simulink model "ZynqBallTrackerFPGA"  (R2017a)
settings: Solver=FixedStepDiscrete  StartTime=0.0  StopTime=5.0  RelTol=1e-3  EnableMultiTasking=on
PostLoadFcn:
  | model_init
values from neighbouring files (symbols this model uses):
  C = 1920    [model_init.m]
  HueTarg = 150    [model_init.m]
  HueTol = 20    [model_init.m]
  Kd = 1    [model_init.m]
  KernG_hdl = reshape(KernG,[],1)    [model_init.m]
  KernR1B2_hdl = reshape(KernR1B2,[],1)    [model_init.m]
  KernR2B1_hdl = reshape(KernR2B1,[],1)    [model_init.m]
  KernRB_hdl = reshape(KernRB,[],1)    [model_init.m]
  Ki = 4    [model_init.m]
  Kp = 16    [model_init.m]
  P = polyfit(u,y,N)    [calc_gamma.m]    (also in model_init.m = calc_gamma(GammaErr,3))
  PWM_CNT = 1024e3    (= 1024000)    [model_init.m]
  R = 1080    [model_init.m]
  SatTarg = 0.38    [model_init.m]
  SatTol = 0.05    [model_init.m]
  SaturationLimit = 256    [model_init.m]
  TsFPGA = TsFr/(R*C)    (= 1.60751028807e-08)    [model_init.m]
  TsFr = 1/FrRt    (= 0.0333333333333)    [model_init.m]
  ValTarg = 170    [model_init.m]
  ValTol = 45    [model_init.m]
undefined symbols (not defined in the file or in its folder): gray, Rec, SDTV
libraries: hdlsllib x51, simulink x12, simulink_need_slupdate x10, visionconversions x2, visiontextngfix x2, visionstatistics x1, dspvision x1, visiongeotforms x1, dspsigattribs x1, dspbuff3 x1
(part 1 of 2)
settings Model: SimulationMode=accelerator  Creator=mfornero  LastModifiedBy=skuznick
settings DataIOCC: LimitDataPoints=on  SaveFormat=Array
settings OptimizationCC: BlockReduction=off  ConditionallyExecuteInputs=off  DefaultParameterBehavior=Inlined  LifeSpan=inf
settings DebuggingCC: AlgebraicLoopMsg=error  UnderspecifiedInitializationDetection=Classic  MergeDetectMultiDrivingBlocksExec=none  InheritedTsInSrcMsg=none  SFUnexpectedBacktrackingDiag=warning  SFNoUnconditionalDefaultTransitionDiag=warning  SFExecutionAtInitializationDiag=none
settings HardwareCC: ProdBitPerPointer=32  ProdBitPerSizeT=32  ProdBitPerPtrDiffT=32  ProdLargestAtomicFloat=None  ProdIntDivRoundTo=Undefined  ProdEndianess=Unspecified  ProdWordSize=32  ProdHWDeviceType=ASIC/FPGA->ASIC/FPGA  ProdEqTarget=off
settings ModelReferenceCC: PropagateSignalLabelsOutOfModel=off
settings GRTTargetCC: TargetLangStandard=C89/C90 (ANSI)  GeneratePreprocessorConditionals=Disable all
settings ConfigComp: CovMetricSettings=dw  CovHtmlReporting=on  CovSaveCumulativeToWorkspaceVar=on  CovSaveSingleToWorkspaceVar=on  CovExternalEMLEnable=off  CovSFcnEnable=off

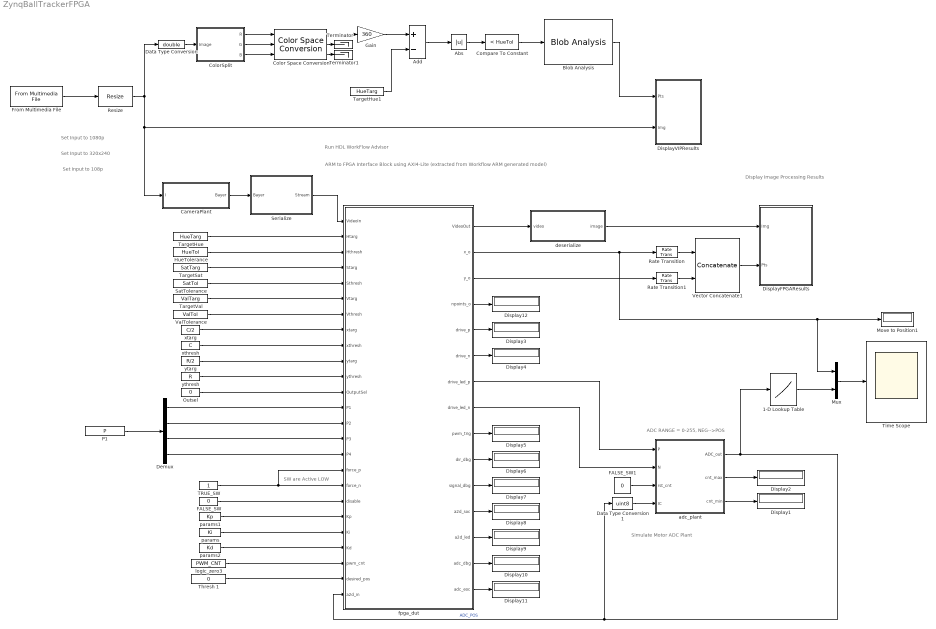
== system ZynqBallTrackerFPGA ==
  note: Set Input to 1080p
  note: Set Input to 320x240
  note: Set Input to 108p
  note: ADC RANGE = 0-255, NEG-->POS
  note: Simulate Motor ADC Plant
  note: Display Image Processing
      | Results
  note: SW are Active LOW
  note: ARM to FPGA Interface Block
      | using AXI4-Lite (extracted from Workflow ARM generated model)
  note: Run HDL WorkFlow
      | Advisor
  1-D Lookup Table : Lookup_n-D  NumberOfTableDimensions=1  BreakpointsForDimension1=[0:1:255]  IndexSearchMethod=Evenly spaced points  Table=[254:-2:-256]  TableDataTypeStr=Inherit: Inherit from 'Table data'  InterpMethod=Flat  DiagnosticForOutOfRangeInput=Error  OutDataTypeStr=fixdt(0,32,0)  RndMeth=Simplest  InputSameDT=on
  Abs : Abs
  Add : Sum  Inputs=+-
  Blob Analysis : visionstatistics/Blob Analysis  Tag=vipblks_row_conv  area=off  centroid=on  bBox=off  majorAxis=off  minorAxis=off  angle=off  eccentricity=off  equivDiameterSq=off  extent=off  perimeter=off  maxBlobs=1  warnIfNumBlobsExceeded=off  isCount=off  useMinArea=on  minArea=100  useMaxArea=off  maxArea=intmax('uint32')  excludeBorderBlob=on  outDT=Specify via Data Types tab  isOutVarDim=off  isFill=off  fillValues=-1  conn=4  isLabel=off  outputMode=Binary point scaling  outputWordLength=16  outputFracLength=0  firstCoeffMode=Binary point scaling  firstCoeffWordLength=16  firstCoeffFracLength=14  secondCoeffMode=Binary point scaling  secondCoeffWordLength=32  secondCoeffFracLength=16  accumMode=Binary point scaling  accumWordLength=32  accumFracLength=0  prodOutputMode=Binary point scaling  prodOutputWordLength=32  prodOutputFracLength=16  roundingMode=Floor  overflowMode=off
      settings: SourceProductName=Computer Vision System Toolbox
  CameraPlant : Subsystem
  Color Space Conversion : visionconversions/Color Space  Conversion  conversion=Obsolete  conversionActive=R'G'B' to HSV  wp_str=D65  rec=Rec. 601 (SDTV)  sys=1125/60/2:1  imagePorts=Separate color signals
      settings: SourceProductName=Computer Vision System Toolbox
  ColorSplit : Subsystem
  Compare To Constant : simulink/Logic and Bit Operations/Compare To Constant  relop=<  const=HueTol  OutDataTypeStr=boolean
  Data Type Conversion : DataTypeConversion  OutDataTypeStr=double
  Data Type Conversion1 : DataTypeConversion  OutDataTypeStr=uint8
  Demux : Demux
  Display{1..12} (12 alike) : Display
  DisplayFPGAResults : Subsystem
  DisplayVIPResults : Subsystem
  FALSE_SW : Constant  Value=0  OutDataTypeStr=boolean  SampleTime=-1
  FALSE_SW1 : Constant  Value=0  OutDataTypeStr=boolean  SampleTime=-1
  From Multimedia File : dspvision/From Multimedia File  inputFilename=Ball.wmv  loop=on  numPlays=inf  outputStreams=Video only  videoDataType=uint8  audioDataType=int16  inheritSampleTime=off  userDefinedSampleTime=TsFr  noAudioOutput=off  isIntensityVideo=off  fourcc=RGB  colorVideoFormat=One multidimensional signal  outputEOF=off  dataOrg=Column-major  audioFrameSize=1024  computeAudioFrameSize=off  outSamplingMode=Frame based
      settings: SourceProductBaseCode=VP
  Gain : Gain  Gain=360
  "HueTolerance " : Constant  Value=HueTol  OutDataTypeStr=Inherit: Inherit via back propagation  SampleTime=-1
  Move to Position1 : Display
  Mux : Mux  Inputs=2
  Outsel : Constant  Value=0  OutDataTypeStr=Inherit: Inherit via back propagation  SampleTime=-1
  P1 : Constant  Value=P  OutDataTypeStr=fixdt(1,25,22)  SampleTime=-1
  Rate Transition : RateTransition  OutPortSampleTime=TsFr
  Rate Transition1 : RateTransition  OutPortSampleTime=TsFr
  Resize : visiongeotforms/Resize  specify=Number of output rows and columns  rfactor=[200 150]  outCols=25  outRows=25  outRowsCols=[R C]  interp_method=Bilinear  antialias=on  useROI=off  roiFlag=off  prodOutputMode=Binary point scaling  prodOutputWordLength=32  prodOutputFracLength=10  roundingMode=Nearest  overflowMode=on
      settings: SourceProductName=Computer Vision System Toolbox  SourceProductBaseCode=VP
  SatTolerance : Constant  Value=SatTol  OutDataTypeStr=Inherit: Inherit via back propagation  SampleTime=-1
  Serialize : Subsystem
  TRUE_SW : Constant  OutDataTypeStr=boolean  SampleTime=-1
  TargetHue : Constant  Value=HueTarg  OutDataTypeStr=Inherit: Inherit via back propagation  SampleTime=-1
  TargetHue1 : Constant  Value=HueTarg  OutDataTypeStr=Inherit: Inherit via back propagation  SampleTime=-1
  TargetSat : Constant  Value=SatTarg  OutDataTypeStr=Inherit: Inherit via back propagation  SampleTime=-1
  TargetVal : Constant  Value=ValTarg  OutDataTypeStr=Inherit: Inherit via back propagation  SampleTime=-1
  Terminator : Terminator
  Terminator1 : Terminator
  Thresh 1 : Constant  Value=0  OutDataTypeStr=Inherit: Inherit via back propagation  SampleTime=-1
  Time Scope : Scope
  ValTolerance : Constant  Value=ValTol  OutDataTypeStr=Inherit: Inherit via back propagation  SampleTime=-1
  Vector Concatenate1 : Concatenate  Mode=Multidimensional array  ConcatenateDimension=2
  adc_plant : Subsystem
  deserialize : Subsystem
  fpga_dut : Subsystem  TreatAsAtomicUnit=on
  logic_zero3 : Constant  Value=PWM_CNT  OutDataTypeStr=fixdt(0,22,0)  SampleTime=-1
  params : Constant  Value=Ki  OutDataTypeStr=fixdt(1,20,14)  SampleTime=-1
  params1 : Constant  Value=Kp  OutDataTypeStr=fixdt(1,20,14)  SampleTime=-1
  params2 : Constant  Value=Kd  OutDataTypeStr=fixdt(1,20,14)  SampleTime=-1
  xtarg : Constant  Value=C/2  OutDataTypeStr=Inherit: Inherit via back propagation  SampleTime=-1
  xthresh : Constant  Value=C  OutDataTypeStr=Inherit: Inherit via back propagation  SampleTime=-1
  ytarg : Constant  Value=R/2  OutDataTypeStr=Inherit: Inherit via back propagation  SampleTime=-1
  ythresh : Constant  Value=R  OutDataTypeStr=Inherit: Inherit via back propagation  SampleTime=-1
  wires:
  From Multimedia File/1 -> Resize/1
  Resize/1 -> CameraPlant/1(I), DisplayVIPResults/2(Img), Data Type Conversion/1
  Blob Analysis/1 -> DisplayVIPResults/1(Pts)
  Data Type Conversion/1 -> ColorSplit/1(Image)
  Serialize/1(Stream) -> fpga_dut/1(VideoIn)
  TargetHue/1 -> fpga_dut/2(Htarg)
  Outsel/1 -> fpga_dut/12(OutputSel)
  "HueTolerance "/1 -> fpga_dut/3(Hthresh)
  fpga_dut/1(VideoOut) -> deserialize/1(video)
  deserialize/1(image) -> DisplayFPGAResults/1(Img)
  ColorSplit/2(G) -> Color Space Conversion/2
  ColorSplit/3(B) -> Color Space Conversion/3
  ColorSplit/1(R) -> Color Space Conversion/1
  Abs/1 -> Compare To Constant/1
  Color Space Conversion/1 -> Gain/1
  Add/1 -> Abs/1
  TargetHue1/1 -> Add/2
  Gain/1 -> Add/1
  Color Space Conversion/2 -> Terminator/1
  Color Space Conversion/3 -> Terminator1/1
  Compare To Constant/1 -> Blob Analysis/1
  Demux/2 -> fpga_dut/14(P2)
  Demux/3 -> fpga_dut/15(P3)
  Demux/1 -> fpga_dut/13(P1)
  Demux/4 -> fpga_dut/16(P4)
  P1/1 -> Demux/1
  CameraPlant/1(Bayer) -> Serialize/1(Bayer)
  TargetSat/1 -> fpga_dut/4(Starg)
  SatTolerance/1 -> fpga_dut/5(Sthresh)
  TargetVal/1 -> fpga_dut/6(Vtarg)
  ValTolerance/1 -> fpga_dut/7(Vthresh)
  adc_plant/2(cnt_max) -> Display2/1
  adc_plant/3(cnt_min) -> Display1/1
  adc_plant/1(ADC_out) -> Data Type Conversion1/1, fpga_dut/25(a2d_in), 1-D Lookup Table/1  "ADC_POS"
  Data Type Conversion1/1 -> adc_plant/4(IC)
  Mux/1 -> Time Scope/1
  fpga_dut/7(drive_led_p) -> adc_plant/1(P)
  fpga_dut/8(drive_led_n) -> adc_plant/2(N)
  FALSE_SW1/1 -> adc_plant/3(rst_cnt)
  1-D Lookup Table/1 -> Mux/2
  fpga_dut/2(x_o) -> Rate Transition/1, Mux/1, Move to Position1/1
  Rate Transition/1 -> Vector Concatenate1/1
  Rate Transition1/1 -> Vector Concatenate1/2
  Vector Concatenate1/1 -> DisplayFPGAResults/2(Pts)
  fpga_dut/3(y_o) -> Rate Transition1/1
  fpga_dut/5(drive_p) -> Display3/1
  fpga_dut/6(drive_n) -> Display4/1
  fpga_dut/9(pwm_trig) -> Display5/1
  fpga_dut/10(dir_dbg) -> Display6/1
  fpga_dut/11(signal_dbg) -> Display7/1
  fpga_dut/12(a2d_soc) -> Display8/1
  fpga_dut/13(a2d_led) -> Display9/1
  fpga_dut/14(adc_dbg) -> Display10/1
  fpga_dut/15(adc_eoc) -> Display11/1
  TRUE_SW/1 -> fpga_dut/17(force_p), fpga_dut/18(force_n)
  FALSE_SW/1 -> fpga_dut/19(disable)
  params/1 -> fpga_dut/21(Ki)
  params1/1 -> fpga_dut/20(Kp)
  params2/1 -> fpga_dut/22(Kd)
  logic_zero3/1 -> fpga_dut/23(pwm_cnt)
  Thresh 1/1 -> fpga_dut/24(desired_pos)
  xtarg/1 -> fpga_dut/8(xtarg)
  xthresh/1 -> fpga_dut/9(xthresh)
  ytarg/1 -> fpga_dut/10(ytarg)
  ythresh/1 -> fpga_dut/11(ythresh)
  fpga_dut/4(npoints_o) -> Display12/1

== system ZynqBallTrackerFPGA/CameraPlant ==
  I : Inport
  Bayer_Phase1 : Constant  Value=3  SampleTime=TsFr
  Gamma Correction VIP : visionconversions/Gamma Correction  operation=De-gamma  gamma=GammaErr  linearSegment=off  breakPoint=0.018
      settings: SourceProductName=Computer Vision System Toolbox  SourceProductBaseCode=VP
  mosaic : MATLAB Function  TreatAsAtomicUnit=on
  Bayer : Outport
  wires:
  Bayer_Phase1/1 -> mosaic/2(phase)
  mosaic/1(Y) -> Bayer/1
  I/1 -> Gamma Correction VIP/1
  Gamma Correction VIP/1 -> mosaic/1(I)

== system ZynqBallTrackerFPGA/ColorSplit ==
  Image : Inport
  SelB : Selector  NumberOfDimensions=3  InputPortWidth=5  IndexOptions=Select all,Select all,Index vector (dialog)  Indices=[1],1,3  OutputSizes=1,1,1
  SelG : Selector  NumberOfDimensions=3  InputPortWidth=5  IndexOptions=Select all,Select all,Index vector (dialog)  Indices=[1],1,2  OutputSizes=1,1,1
  SelR : Selector  NumberOfDimensions=3  InputPortWidth=5  IndexOptions=Select all,Select all,Index vector (dialog)  Indices=[1],1,1  OutputSizes=1,1,1
  R : Outport
  G : Outport  Port=2
  B : Outport  Port=3
  wires:
  SelR/1 -> R/1
  SelG/1 -> G/1
  Image/1 -> SelB/1, SelR/1, SelG/1
  SelB/1 -> B/1

== system ZynqBallTrackerFPGA/DisplayFPGAResults ==
  Img : Inport
  Pts : Inport  Port=2
  Draw Markers : visiontextngfix/Draw Markers  shape=Circle  size=msize  fill=on  fillClrSource=Specify via dialog  display=User-specified value  intensity=200  color=[255 0 0]  opacity=1.0  viewport=Entire image  antialiasing=off  inType=Obsolete  imagePorts=One multidimensional signal  prodOutputMode=Binary point scaling  prodOutputWordLength=32  prodOutputFracLength=14  memoryMode=Specify word length  memoryWordLength=16  memoryFracLength=14  roundingMode=Floor  overflowMode=off
      settings: SourceProductName=Computer Vision System Toolbox  SourceProductBaseCode=VP
  FPGAViewer : VideoViewer  colormapValue=gray(256)  FigPos=[562 1008 521 308]
  wires:
  Img/1 -> Draw Markers/1
  Pts/1 -> Draw Markers/2
  Draw Markers/1 -> FPGAViewer/1

== system ZynqBallTrackerFPGA/DisplayVIPResults ==
  Pts : Inport
  Img : Inport  Port=2
  Draw Markers : visiontextngfix/Draw Markers  shape=Circle  size=msize  fill=on  fillClrSource=Specify via dialog  display=User-specified value  intensity=200  color=[255 0 0]  opacity=1.0  viewport=Entire image  antialiasing=off  inType=Obsolete  imagePorts=One multidimensional signal  prodOutputMode=Binary point scaling  prodOutputWordLength=32  prodOutputFracLength=14  memoryMode=Specify word length  memoryWordLength=16  memoryFracLength=14  roundingMode=Floor  overflowMode=off
      settings: SourceProductName=Computer Vision System Toolbox  SourceProductBaseCode=VP
  VIPViewer : VideoViewer  colormapValue=gray(256)  FigPos=[44 1004 496 307]
  wires:
  Draw Markers/1 -> VIPViewer/1
  Pts/1 -> Draw Markers/2
  Img/1 -> Draw Markers/1

== system ZynqBallTrackerFPGA/Serialize ==
  Bayer : Inport
  Convert 2-D to 1-D : dspsigattribs/Convert 2-D to 1-D
      settings: SourceProductName=DSP System Toolbox  SourceProductBaseCode=DS
  Frame Conversion : FrameConversion  InheritSamplingMode=off
  G : Constant  Value=zeros(R,C)  OutDataTypeStr=uint8  SampleTime=TsFr
  R : Constant  Value=zeros(R,C)  OutDataTypeStr=uint8  SampleTime=TsFr
  RGB_to_RGB32 : MATLAB Function  TreatAsAtomicUnit=on
  Unbuffer : Unbuffer
  Stream : Outport
  wires:
  Convert 2-D to 1-D/1 -> Frame Conversion/1
  RGB_to_RGB32/1(RGB32) -> Convert 2-D to 1-D/1
  Frame Conversion/1 -> Unbuffer/1
  Unbuffer/1 -> Stream/1
  Bayer/1 -> RGB_to_RGB32/3(B)
  R/1 -> RGB_to_RGB32/1(R)
  G/1 -> RGB_to_RGB32/2(G)

== system ZynqBallTrackerFPGA/adc_plant ==
  P : Inport
  N : Inport  Port=2
  rst_cnt : Inport  Port=3
  IC : Inport  Port=4
  Compare To Constant : simulink/Logic and Bit Operations/Compare To Constant  relop===  const=255  OutDataTypeStr=boolean
  Compare To Constant1 : simulink/Logic and Bit Operations/Compare To Constant  relop===  const=0  OutDataTypeStr=boolean
  Constant : Constant  OutDataTypeStr=boolean  SampleTime=-1
  Constant1 : Constant  Value=0  OutDataTypeStr=boolean  SampleTime=-1
  Delay : Delay  DelayLength=1  InitialCondition=1
  HDL Counter : hdlsllib/HDL Operations/HDL Counter  CountType=Free running  CountInit=0  CountStep=1  CountMax=255  CountFromType=Initial value  CountFrom=0  CountResetPort=on  CountLoadPort=on  CountEnbPort=on  CountDirPort=on  CountDataType=Unsigned  CountWordLen=8  CountFracLen=0  CountSampTime=-1
      settings: SourceProductName=HDL Coder  SourceProductBaseCode=HD
  Logical Operator1 : Logic  IconShape=distinctive  AllPortsSameDT=off  OutDataTypeStr=boolean
  Logical Operator2 : Logic  IconShape=distinctive  AllPortsSameDT=off  OutDataTypeStr=boolean
  Logical Operator4 : Logic  Operator=OR  IconShape=distinctive  AllPortsSameDT=off  OutDataTypeStr=boolean
  Switch : Switch  Criteria=u2 ~= 0
  Switch1 : Switch  Criteria=u2 ~= 0
  ADC_out : Outport
  cnt_max : Outport  Port=2
  cnt_min : Outport  Port=3
  wires:
  Logical Operator2/1 -> Logical Operator1/2
  Switch1/1 -> Logical Operator2/2
  Switch/1 -> Logical Operator2/1
  HDL Counter/1 -> Compare To Constant1/1, Compare To Constant/1, ADC_out/1
  P/1 -> HDL Counter/5, Switch1/1, Logical Operator4/1
  N/1 -> Switch/1, Logical Operator4/2
  rst_cnt/1 -> HDL Counter/1
  Compare To Constant/1 -> Switch/2, cnt_max/1
  Compare To Constant1/1 -> Switch1/2, cnt_min/1
  Constant/1 -> Switch1/3, Switch/3
  Logical Operator1/1 -> HDL Counter/4
  Logical Operator4/1 -> Logical Operator1/1
  IC/1 -> HDL Counter/3
  Constant1/1 -> Delay/1
  Delay/1 -> HDL Counter/2

== system ZynqBallTrackerFPGA/deserialize ==
  video : Inport
  RGB32_to_RGB : MATLAB Function  TreatAsAtomicUnit=on  mask(RGB32 to RGB){doTranspose=on}
      mask prompts: doTranspose "Transpose Data"
      mask help: Convert from Packed RGB (uint32) to Planar RGB (uint8)
  Rate Transition : RateTransition  OutPortSampleTime=TsFr
  Reshape : Reshape  OutputDimensionality=Customize  OutputDimensions=[C,R]
  Unit Delay Enabled : simulink_need_slupdate/Unit Delay Enabled  vinit=0.0  tsamp=-1
      settings: SourceProductName=Simulink  SourceProductBaseCode=SL
  buffer : Subsystem
  get_sof : Subsystem
  image : Outport
  wires:
  Rate Transition/1 -> Reshape/1
  video/1 -> get_sof/1(Video), buffer/1(stream)
  Reshape/1 -> RGB32_to_RGB/1(RGB32)
  buffer/1(buff) -> Unit Delay Enabled/1
  Unit Delay Enabled/1 -> Rate Transition/1
  get_sof/1(SoF) -> Unit Delay Enabled/2
  RGB32_to_RGB/1(RGB) -> image/1

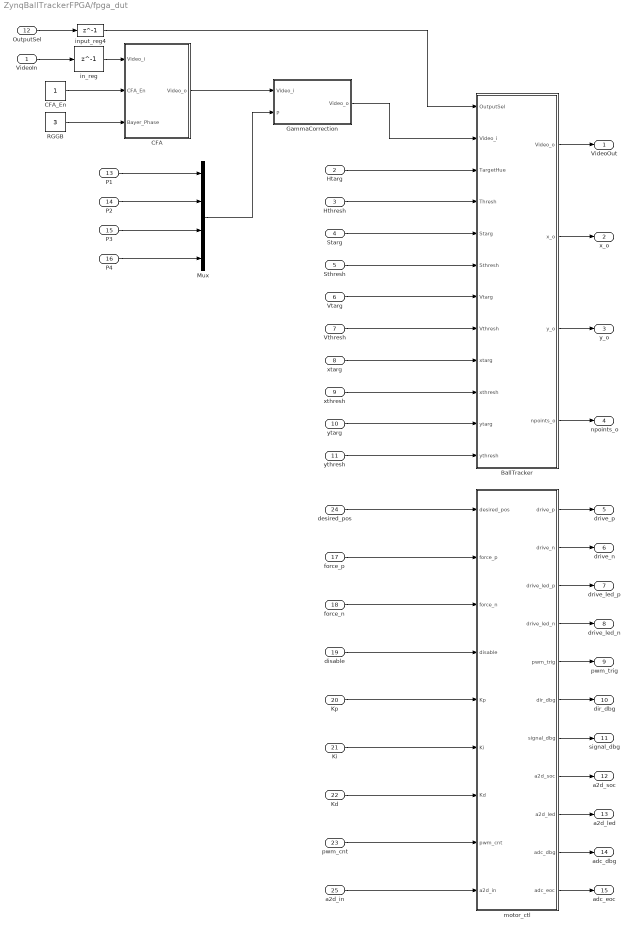
== system ZynqBallTrackerFPGA/fpga_dut ==
  VideoIn : Inport  OutDataTypeStr=uint32
  Htarg : Inport  Port=2  OutDataTypeStr=fixdt(0,9,0)
  Hthresh : Inport  Port=3  OutDataTypeStr=fixdt(0,9,0)
  Starg : Inport  Port=4  OutDataTypeStr=fixdt(0,16,15)
  Sthresh : Inport  Port=5  OutDataTypeStr=fixdt(0,16,15)
  Vtarg : Inport  Port=6  OutDataTypeStr=fixdt(0,8,0)
  Vthresh : Inport  Port=7  OutDataTypeStr=fixdt(0,8,0)
  xtarg : Inport  Port=8
  xthresh : Inport  Port=9
  ytarg : Inport  Port=10
  ythresh : Inport  Port=11
  OutputSel : Inport  Port=12  OutDataTypeStr=fixdt(0,3,0)
  P1 : Inport  Port=13  OutDataTypeStr=fixdt(1,25,22)
  P2 : Inport  Port=14  OutDataTypeStr=fixdt(1,25,22)
  P3 : Inport  Port=15  OutDataTypeStr=fixdt(1,25,22)
  P4 : Inport  Port=16  OutDataTypeStr=fixdt(1,25,22)
  force_p : Inport  Port=17  OutDataTypeStr=boolean
  force_n : Inport  Port=18  OutDataTypeStr=boolean
  disable : Inport  Port=19
  Kp : Inport  Port=20
  Ki : Inport  Port=21
  Kd : Inport  Port=22
  pwm_cnt : Inport  Port=23
  desired_pos : Inport  Port=24  OutDataTypeStr=fixdt(1, 9, 0)
  a2d_in : Inport  Port=25
  BallTracker : Subsystem
      settings: AttributesFormatString=|
      | ----------
      | op:1
      | ip:1
  CFA : Subsystem
  CFA_En : Constant  OutDataTypeStr=boolean  SampleTime=-1
  GammaCorrection : Subsystem
      settings: AttributesFormatString=|
      | ----------
      | op:1
      | ip:1
  Mux : Mux
  RGGB : Constant  Value=3  OutDataTypeStr=fixdt(0,2,0)  SampleTime=-1
  in_reg : Delay  DelayLength=1  InitialCondition=0  UseCircularBuffer=on
  input_reg4 : Delay  DelayLength=1  InitialCondition=0  UseCircularBuffer=on
  motor_ctl : Subsystem
  VideoOut : Outport
  x_o : Outport  Port=2
  y_o : Outport  Port=3
  npoints_o : Outport  Port=4
  drive_p : Outport  Port=5
  drive_n : Outport  Port=6
  drive_led_p : Outport  Port=7
  drive_led_n : Outport  Port=8
  pwm_trig : Outport  Port=9
  dir_dbg : Outport  Port=10
  signal_dbg : Outport  Port=11
  a2d_soc : Outport  Port=12
  a2d_led : Outport  Port=13
  adc_dbg : Outport  Port=14
  adc_eoc : Outport  Port=15
  wires:
  VideoIn/1 -> in_reg/1
  OutputSel/1 -> input_reg4/1
  in_reg/1 -> CFA/1(Video_i)
  RGGB/1 -> CFA/3(Bayer_Phase)
  CFA_En/1 -> CFA/2(CFA_En)
  input_reg4/1 -> BallTracker/1(OutputSel)
  Htarg/1 -> BallTracker/3(TargetHue)
  BallTracker/1(Video_o) -> VideoOut/1
  BallTracker/2(x_o) -> x_o/1
  BallTracker/3(y_o) -> y_o/1
  Hthresh/1 -> BallTracker/4(Thresh)
  P1/1 -> Mux/1
  P3/1 -> Mux/3
  P4/1 -> Mux/4
  P2/1 -> Mux/2
  CFA/1(Video_o) -> GammaCorrection/1(Video_i)
  GammaCorrection/1(Video_o) -> BallTracker/2(Video_i)
  Mux/1 -> GammaCorrection/2(P)
  Vtarg/1 -> BallTracker/7(Vtarg)
  Starg/1 -> BallTracker/5(Starg)
  Sthresh/1 -> BallTracker/6(Sthresh)
  Vthresh/1 -> BallTracker/8(Vthresh)
  force_p/1 -> motor_ctl/2(force_p)
  force_n/1 -> motor_ctl/3(force_n)
  disable/1 -> motor_ctl/4(disable)
  Kp/1 -> motor_ctl/5(Kp)
  Ki/1 -> motor_ctl/6(Ki)
  Kd/1 -> motor_ctl/7(Kd)
  pwm_cnt/1 -> motor_ctl/8(pwm_cnt)
  a2d_in/1 -> motor_ctl/9(a2d_in)
  motor_ctl/1(drive_p) -> drive_p/1
  motor_ctl/2(drive_n) -> drive_n/1
  motor_ctl/3(drive_led_p) -> drive_led_p/1
  motor_ctl/4(drive_led_n) -> drive_led_n/1
  motor_ctl/5(pwm_trig) -> pwm_trig/1
  motor_ctl/6(dir_dbg) -> dir_dbg/1
  motor_ctl/7(signal_dbg) -> signal_dbg/1
  motor_ctl/8(a2d_soc) -> a2d_soc/1
  motor_ctl/9(a2d_led) -> a2d_led/1
  motor_ctl/10(adc_dbg) -> adc_dbg/1
  motor_ctl/11(adc_eoc) -> adc_eoc/1
  desired_pos/1 -> motor_ctl/1(desired_pos)
  xtarg/1 -> BallTracker/9(xtarg)
  xthresh/1 -> BallTracker/10(xthresh)
  ytarg/1 -> BallTracker/11(ytarg)
  ythresh/1 -> BallTracker/12(ythresh)
  BallTracker/4(npoints_o) -> npoints_o/1

== system ZynqBallTrackerFPGA/deserialize/buffer ==
  stream : Inport
  Delay Line : dspbuff3/Delay Line  siz=R*C  ic=0  directfeed=off  enable_output=off  hold_output=on  OutputFrames=on
      settings: SourceProductName=DSP System Toolbox  SourceProductBaseCode=DS
  Frame Conversion : FrameConversion  InheritSamplingMode=off  OutFrame=Sample-based
  buff : Outport
  wires:
  stream/1 -> Delay Line/1
  Delay Line/1 -> Frame Conversion/1
  Frame Conversion/1 -> buff/1

== system ZynqBallTrackerFPGA/deserialize/get_sof ==
  Video : Inport
  Bit Slice : hdlsllib/HDL Operations/Bit Slice  lidx=31  ridx=31
      settings: SourceProductName=HDL Coder  SourceProductBaseCode=HD
  Data Type Conversion : DataTypeConversion  OutDataTypeStr=boolean
  SoF : Outport
  wires:
  Bit Slice/1 -> Data Type Conversion/1
  Video/1 -> Bit Slice/1
  Data Type Conversion/1 -> SoF/1

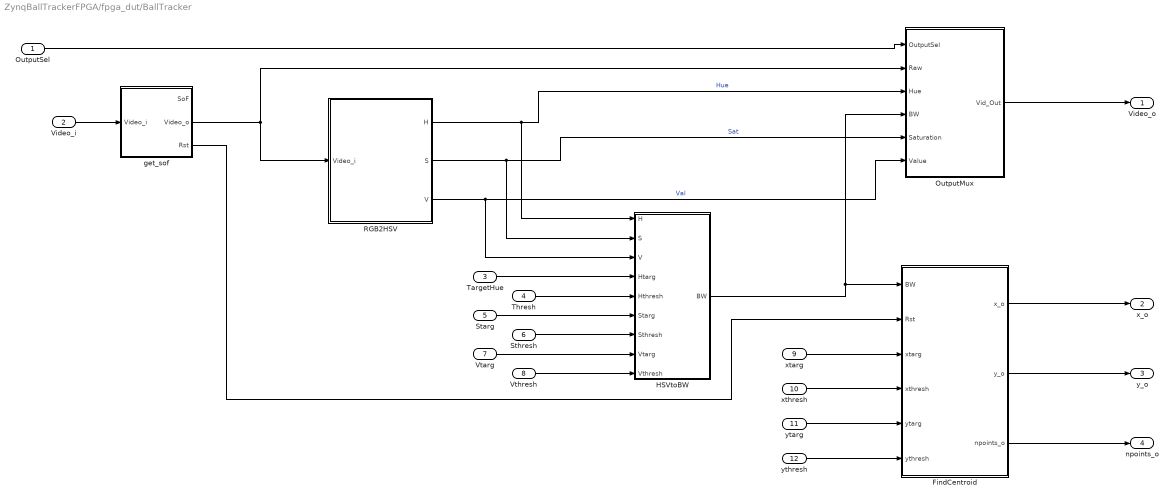
== system ZynqBallTrackerFPGA/fpga_dut/BallTracker ==
  OutputSel : Inport
  Video_i : Inport  Port=2
  TargetHue : Inport  Port=3
  Thresh : Inport  Port=4
  Starg : Inport  Port=5
  Sthresh : Inport  Port=6
  Vtarg : Inport  Port=7
  Vthresh : Inport  Port=8
  xtarg : Inport  Port=9
  xthresh : Inport  Port=10
  ytarg : Inport  Port=11
  ythresh : Inport  Port=12
  FindCentroid : Subsystem
  HSVtoBW : Subsystem
  OutputMux : Subsystem
      settings: AttributesFormatString=|
      | ----------
      | op:1
      | ip:1
      | dp:on
  RGB2HSV : Subsystem
  get_sof : Subsystem
      settings: AttributesFormatString=|
      | ----------
      | ip:1
  Video_o : Outport
  x_o : Outport  Port=2
  y_o : Outport  Port=3
  npoints_o : Outport  Port=4
  wires:
  OutputSel/1 -> OutputMux/1(OutputSel)
  RGB2HSV/1(H) -> HSVtoBW/1(H), OutputMux/3(Hue)  "Hue"
  FindCentroid/1(x_o) -> x_o/1
  FindCentroid/2(y_o) -> y_o/1
  OutputMux/1(Vid_Out) -> Video_o/1
  RGB2HSV/3(V) -> HSVtoBW/3(V), OutputMux/6(Value)  "Val"
  RGB2HSV/2(S) -> HSVtoBW/2(S), OutputMux/5(Saturation)  "Sat"
  HSVtoBW/1(BW) -> FindCentroid/1(BW), OutputMux/4(BW)
  TargetHue/1 -> HSVtoBW/4(Htarg)
  Thresh/1 -> HSVtoBW/5(Hthresh)
  Starg/1 -> HSVtoBW/6(Starg)
  Sthresh/1 -> HSVtoBW/7(Sthresh)
  Vtarg/1 -> HSVtoBW/8(Vtarg)
  Vthresh/1 -> HSVtoBW/9(Vthresh)
  Video_i/1 -> get_sof/1(Video_i)
  get_sof/2(Video_o) -> RGB2HSV/1(Video_i), OutputMux/2(Raw)
  get_sof/3(Rst) -> FindCentroid/2(Rst)
  xthresh/1 -> FindCentroid/4(xthresh)
  ytarg/1 -> FindCentroid/5(ytarg)
  xtarg/1 -> FindCentroid/3(xtarg)
  ythresh/1 -> FindCentroid/6(ythresh)
  FindCentroid/3(npoints_o) -> npoints_o/1

== system ZynqBallTrackerFPGA/fpga_dut/CFA ==
  note: HDL Implementation o f Demosaicing with The Bayer Pattern
      | Based on http://www.unc.edu/~rjean/demosaicing/demosaicing.pdf
  Video_i : Inport
  CFA_En : Inport  Port=2  OutDataTypeStr=boolean
  Bayer_Phase : Inport  Port=3  OutDataTypeStr=fixdt(0,2,0)
  MW_CFA : Subsystem
  Video_o : Outport
  wires:
  Video_i/1 -> MW_CFA/1(Video_i)
  CFA_En/1 -> MW_CFA/2(CFA_En)
  Bayer_Phase/1 -> MW_CFA/3(Bayer_Phase)
  MW_CFA/1(Video_o) -> Video_o/1

== system ZynqBallTrackerFPGA/fpga_dut/GammaCorrection ==
  Video_i : Inport
  P : Inport  Port=2
  Gama CorrectionCore : Subsystem
  RGB_to_Vid : Subsystem
  Vid_to_RGB : Subsystem
  Video_o : Outport
  wires:
  RGB_to_Vid/1(Video_o) -> Video_o/1
  Gama CorrectionCore/3(B_o) -> RGB_to_Vid/4(B)
  Gama CorrectionCore/2(G_o) -> RGB_to_Vid/3(G)
  Gama CorrectionCore/1(R_o) -> RGB_to_Vid/2(R)
  Vid_to_RGB/1(SoF_o) -> RGB_to_Vid/1(SoF)
  Vid_to_RGB/4(B_o) -> Gama CorrectionCore/3(B_i)
  Vid_to_RGB/3(G_o) -> Gama CorrectionCore/2(G_i)
  Vid_to_RGB/2(R_o) -> Gama CorrectionCore/1(R_i)
  Video_i/1 -> Vid_to_RGB/1(Video_i)
  P/1 -> Gama CorrectionCore/4(P)

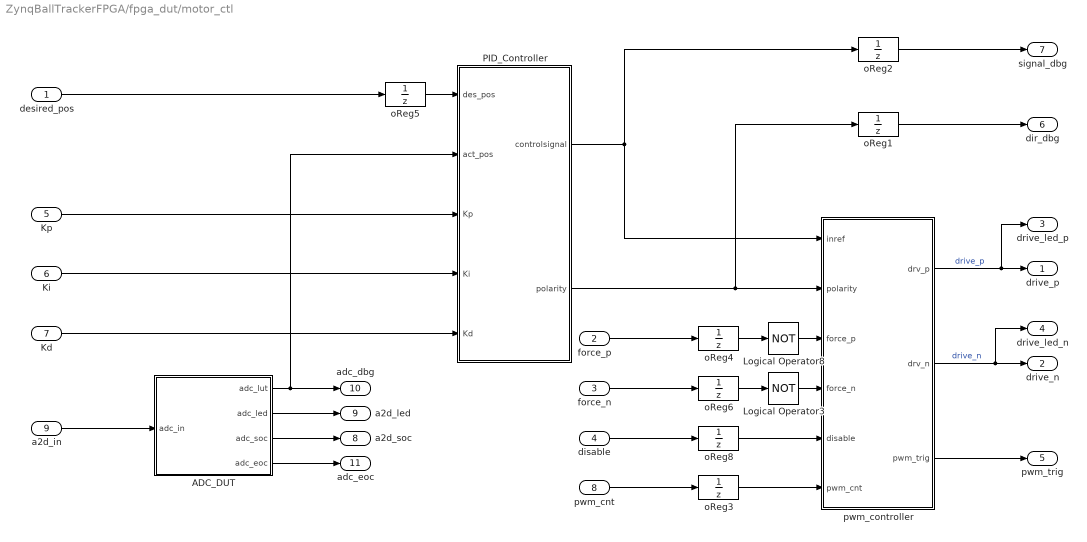
== system ZynqBallTrackerFPGA/fpga_dut/motor_ctl ==
  desired_pos : Inport
  force_p : Inport  Port=2  OutDataTypeStr=boolean
  force_n : Inport  Port=3  OutDataTypeStr=boolean
  disable : Inport  Port=4
  Kp : Inport  Port=5
  Ki : Inport  Port=6
  Kd : Inport  Port=7
  pwm_cnt : Inport  Port=8
  a2d_in : Inport  Port=9
  ADC_DUT : Subsystem  SystemSampleTime=2e-8
  Logical Operator3 : Logic  Operator=NOT  IconShape=distinctive  AllPortsSameDT=off  OutDataTypeStr=boolean
  Logical Operator8 : Logic  Operator=NOT  IconShape=distinctive  AllPortsSameDT=off  OutDataTypeStr=boolean
  PID_Controller : Subsystem  TreatAsAtomicUnit=on  SystemSampleTime=TsFPGA
  oReg{1..6,8} (7 alike) : UnitDelay  SampleTime=-1
  pwm_controller : Subsystem  TreatAsAtomicUnit=on
  drive_p : Outport
  drive_n : Outport  Port=2
  drive_led_p : Outport  Port=3
  drive_led_n : Outport  Port=4
  pwm_trig : Outport  Port=5
  dir_dbg : Outport  Port=6
  signal_dbg : Outport  Port=7
  a2d_soc : Outport  Port=8
  a2d_led : Outport  Port=9
  adc_dbg : Outport  Port=10
  adc_eoc : Outport  Port=11
  wires:
  pwm_controller/1(drv_p) -> drive_led_p/1, drive_p/1  "drive_p"
  pwm_controller/2(drv_n) -> drive_led_n/1, drive_n/1  "drive_n"
  Logical Operator8/1 -> pwm_controller/3(force_p)
  Logical Operator3/1 -> pwm_controller/4(force_n)
  oReg4/1 -> Logical Operator8/1
  oReg6/1 -> Logical Operator3/1
  a2d_in/1 -> ADC_DUT/1(adc_in)
  oReg2/1 -> signal_dbg/1
  oReg1/1 -> dir_dbg/1
  ADC_DUT/1(adc_lut) -> adc_dbg/1, PID_Controller/2(act_pos)
  oReg8/1 -> pwm_controller/5(disable)
  pwm_controller/3(pwm_trig) -> pwm_trig/1
  PID_Controller/2(polarity) -> oReg1/1, pwm_controller/2(polarity)
  PID_Controller/1(controlsignal) -> oReg2/1, pwm_controller/1(inref)
  force_n/1 -> oReg6/1
  force_p/1 -> oReg4/1
  disable/1 -> oReg8/1
  ADC_DUT/4(adc_eoc) -> adc_eoc/1
  ADC_DUT/3(adc_soc) -> a2d_soc/1
  ADC_DUT/2(adc_led) -> a2d_led/1
  Kp/1 -> PID_Controller/3(Kp)
  Ki/1 -> PID_Controller/4(Ki)
  Kd/1 -> PID_Controller/5(Kd)
  oReg3/1 -> pwm_controller/6(pwm_cnt)
  pwm_cnt/1 -> oReg3/1
  oReg5/1 -> PID_Controller/1(des_pos)
  desired_pos/1 -> oReg5/1

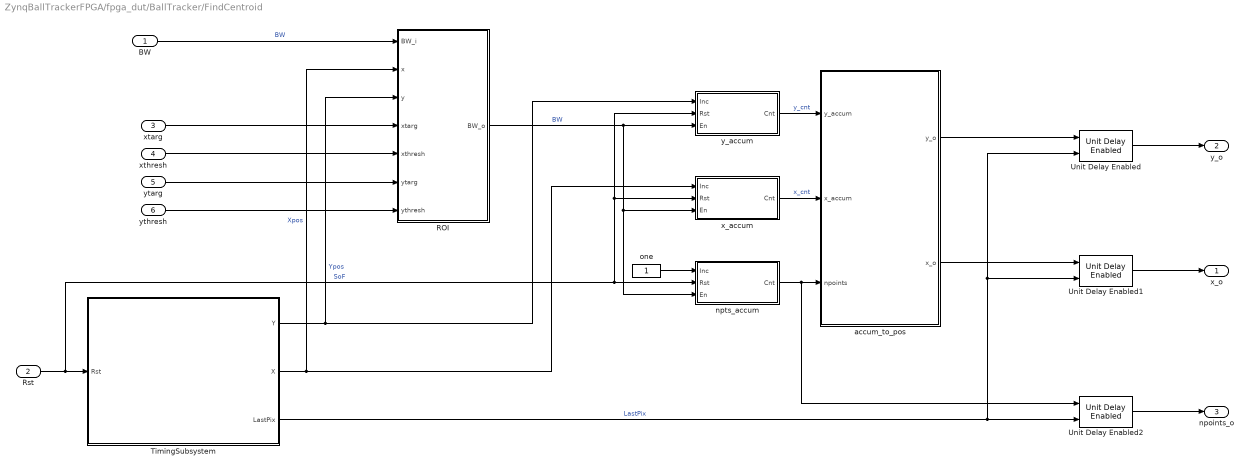
== system ZynqBallTrackerFPGA/fpga_dut/BallTracker/FindCentroid ==
  BW : Inport
  Rst : Inport  Port=2
  xtarg : Inport  Port=3
  xthresh : Inport  Port=4
  ytarg : Inport  Port=5
  ythresh : Inport  Port=6
  ROI : Subsystem
  TimingSubsystem : Subsystem
  Unit Delay Enabled : simulink_need_slupdate/Unit Delay Enabled  vinit=fi(0,0,32,0)  tsamp=-1
      settings: SourceProductName=Simulink  SourceProductBaseCode=SL
  Unit Delay Enabled1 : simulink_need_slupdate/Unit Delay Enabled  vinit=fi(0,0,32,0)  tsamp=-1
      settings: SourceProductName=Simulink  SourceProductBaseCode=SL
  Unit Delay Enabled2 : simulink_need_slupdate/Unit Delay Enabled  vinit=fi(0,0,32,0)  tsamp=-1
      settings: SourceProductName=Simulink  SourceProductBaseCode=SL
  accum_to_pos : Subsystem
  npts_accum : Subsystem  mask(Accumulator){MaxVal=R*C/8}
      mask prompts: MaxVal "Accumulator Maximum Value"
      mask help: Accumulate values
      settings: AttributesFormatString=|
      | ----------
      | ip:1
  one : Constant  OutDataTypeStr=Inherit: Inherit via back propagation  SampleTime=TsFPGA
  x_accum : Subsystem  mask(Accumulator){MaxVal=max(R-1,C-1)*R*C}
      mask prompts: MaxVal "Accumulator Maximum Value"
      mask help: Accumulate values
      settings: AttributesFormatString=|
      | ----------
      | ip:1
  y_accum : Subsystem  mask(Accumulator){MaxVal=max(R-1,C-1)*R*C}
      mask prompts: MaxVal "Accumulator Maximum Value"
      mask help: Accumulate values
      settings: AttributesFormatString=|
      | ----------
      | ip:1
  x_o : Outport
  y_o : Outport  Port=2
  npoints_o : Outport  Port=3
  wires:
  Rst/1 -> y_accum/2(Rst), x_accum/2(Rst), npts_accum/2(Rst), TimingSubsystem/1(Rst)  "SoF"
  ROI/1(BW_o) -> npts_accum/3(En), x_accum/3(En), y_accum/3(En)  "BW"
  TimingSubsystem/2(X) -> ROI/2(x), x_accum/1(Inc)  "Xpos"
  TimingSubsystem/1(Y) -> ROI/3(y), y_accum/1(Inc)  "Ypos"
  one/1 -> npts_accum/1(Inc)
  TimingSubsystem/3(LastPix) -> Unit Delay Enabled2/2, Unit Delay Enabled/2, Unit Delay Enabled1/2  "LastPix"
  y_accum/1(Cnt) -> accum_to_pos/1(y_accum)  "y_cnt"
  x_accum/1(Cnt) -> accum_to_pos/2(x_accum)  "x_cnt"
  npts_accum/1(Cnt) -> Unit Delay Enabled2/1, accum_to_pos/3(npoints)
  accum_to_pos/1(y_o) -> Unit Delay Enabled/1
  Unit Delay Enabled/1 -> y_o/1
  accum_to_pos/2(x_o) -> Unit Delay Enabled1/1
  Unit Delay Enabled1/1 -> x_o/1
  BW/1 -> ROI/1(BW_i)  "BW"
  xthresh/1 -> ROI/5(xthresh)
  ytarg/1 -> ROI/6(ytarg)
  xtarg/1 -> ROI/4(xtarg)
  ythresh/1 -> ROI/7(ythresh)
  Unit Delay Enabled2/1 -> npoints_o/1

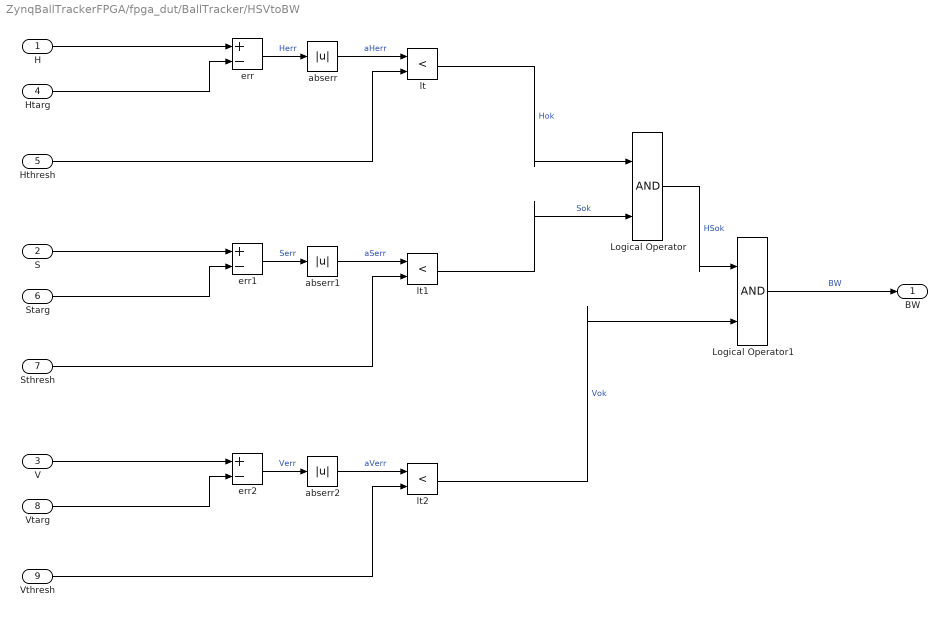
== system ZynqBallTrackerFPGA/fpga_dut/BallTracker/HSVtoBW ==
  H : Inport
  S : Inport  Port=2
  V : Inport  Port=3
  Htarg : Inport  Port=4
  Hthresh : Inport  Port=5
  Starg : Inport  Port=6
  Sthresh : Inport  Port=7
  Vtarg : Inport  Port=8
  Vthresh : Inport  Port=9
  Logical Operator : Logic  IconShape=distinctive  AllPortsSameDT=off  OutDataTypeStr=boolean
      settings: AttributesFormatString=|
      | ----------
      | op:1
  Logical Operator1 : Logic  IconShape=distinctive  AllPortsSameDT=off  OutDataTypeStr=boolean
      settings: AttributesFormatString=|
      | ----------
      | op:1
  abserr : Abs
  abserr1 : Abs
  abserr2 : Abs
  err : Sum  Inputs=+-
      settings: AttributesFormatString=|
      | ----------
      | op:1
      | ip:1
  err1 : Sum  Inputs=+-
      settings: AttributesFormatString=|
      | ----------
      | op:1
      | ip:1
  err2 : Sum  Inputs=+-
      settings: AttributesFormatString=|
      | ----------
      | op:1
      | ip:1
  lt : RelationalOperator  Operator=<  OutDataTypeStr=boolean  RndMeth=Nearest
      settings: AttributesFormatString=|
      | ----------
      | op:1
      | ip:1
  lt1 : RelationalOperator  Operator=<  OutDataTypeStr=boolean  RndMeth=Nearest
      settings: AttributesFormatString=|
      | ----------
      | op:1
      | ip:1
  lt2 : RelationalOperator  Operator=<  OutDataTypeStr=boolean  RndMeth=Nearest
      settings: AttributesFormatString=|
      | ----------
      | op:1
      | ip:1
  BW : Outport
  wires:
  Htarg/1 -> err/2
  err/1 -> abserr/1  "Herr"
  abserr/1 -> lt/1  "aHerr"
  Hthresh/1 -> lt/2
  lt/1 -> Logical Operator/1  "Hok"
  H/1 -> err/1
  Starg/1 -> err1/2
  err1/1 -> abserr1/1  "Serr"
  abserr1/1 -> lt1/1  "aSerr"
  Sthresh/1 -> lt1/2
  S/1 -> err1/1
  lt1/1 -> Logical Operator/2  "Sok"
  Logical Operator/1 -> Logical Operator1/1  "HSok"
  Logical Operator1/1 -> BW/1  "BW"
  Vtarg/1 -> err2/2
  err2/1 -> abserr2/1  "Verr"
  abserr2/1 -> lt2/1  "aVerr"
  Vthresh/1 -> lt2/2
  V/1 -> err2/1
  lt2/1 -> Logical Operator1/2  "Vok"

== system ZynqBallTrackerFPGA/fpga_dut/BallTracker/OutputMux ==
  OutputSel : Inport
  Raw : Inport  Port=2
  Hue : Inport  Port=3
  BW : Inport  Port=4
  Saturation : Inport  Port=5
  Value : Inport  Port=6
  HuetoRGB : Subsystem
      settings: AttributesFormatString=|
      | ----------
      | dp:on
  Multiport Switch : MultiPortSwitch  DataPortOrder=Zero-based contiguous  Inputs=8  DiagnosticForDefault=None
      settings: AttributesFormatString=|
      | ----------
      | op:2
      | ip:1
  SattoRGB2 : Subsystem
      settings: AttributesFormatString=|
      | ----------
      | dp:on
  Switch : Switch  Criteria=u2 ~= 0
      settings: AttributesFormatString=|
      | ----------
      | op:1
  Y2RGB : Subsystem
  Y2RGB1 : Subsystem
  black : Constant  Value=0  OutDataTypeStr=uint8  SampleTime=-1
  black1 : Constant  Value=0  OutDataTypeStr=uint8  SampleTime=-1
  white : Constant  Value=255  OutDataTypeStr=uint8  SampleTime=-1
  Vid_Out : Outport
  wires:
  Raw/1 -> Multiport Switch/2
  Y2RGB1/1(Video_Out) -> Multiport Switch/4
  BW/1 -> Switch/2
  Multiport Switch/1 -> Vid_Out/1
  black/1 -> Switch/3
  white/1 -> Switch/1
  Switch/1 -> Y2RGB1/1(Y_i)
  Hue/1 -> HuetoRGB/1(Hue)
  HuetoRGB/1(RGB) -> Multiport Switch/3
  OutputSel/1 -> Multiport Switch/1
  Y2RGB/1(Video_Out) -> Multiport Switch/6
  black1/1 -> Multiport Switch/9, Multiport Switch/8, Multiport Switch/7
  Saturation/1 -> SattoRGB2/1(Sat)
  Value/1 -> Y2RGB/1(Y_i)
  SattoRGB2/1(RGB) -> Multiport Switch/5

== system ZynqBallTrackerFPGA/fpga_dut/BallTracker/RGB2HSV ==
  Video_i : Inport
  Blue : hdlsllib/HDL Operations/Bit Slice  lidx=7  ridx=0
      settings: SourceProductName=HDL Coder  SourceProductBaseCode=HD
  Green : hdlsllib/HDL Operations/Bit Slice  lidx=15  ridx=8
      settings: SourceProductName=HDL Coder  SourceProductBaseCode=HD
  RGBtoHue : Subsystem
      settings: AttributesFormatString=|
      | ----------
      | op:1
      | ip:1
      | dp:on
  Red : hdlsllib/HDL Operations/Bit Slice  lidx=23  ridx=16
      settings: SourceProductName=HDL Coder  SourceProductBaseCode=HD
  H : Outport
  S : Outport  Port=2
  V : Outport  Port=3
  wires:
  Video_i/1 -> Red/1, Green/1, Blue/1
  Red/1 -> RGBtoHue/1(R)  "R"
  Green/1 -> RGBtoHue/2(G)  "G"
  Blue/1 -> RGBtoHue/3(B)  "B"
  RGBtoHue/1(Hue) -> H/1
  RGBtoHue/3(Value) -> V/1
  RGBtoHue/2(Saturation) -> S/1

== system ZynqBallTrackerFPGA/fpga_dut/BallTracker/get_sof ==
  Video_i : Inport
  Bit Slice : hdlsllib/HDL Operations/Bit Slice  lidx=31  ridx=31
      settings: SourceProductName=HDL Coder  SourceProductBaseCode=HD
  Data Type Conversion : DataTypeConversion  OutDataTypeStr=boolean
  Delay1 : Delay  DelayLength=1
  Delay2 : Delay  DelayLength=1
  SoF : Outport
  Video_o : Outport  Port=2
  Rst : Outport  Port=3
  wires:
  Bit Slice/1 -> Data Type Conversion/1
  Video_i/1 -> Delay2/1, Bit Slice/1
  Data Type Conversion/1 -> Rst/1, Delay1/1
  Delay2/1 -> Video_o/1
  Delay1/1 -> SoF/1

== system ZynqBallTrackerFPGA/fpga_dut/CFA/MW_CFA ==
  Video_i : Inport
  CFA_En : Inport  Port=2  OutDataTypeStr=boolean
  Bayer_Phase : Inport  Port=3  OutDataTypeStr=fixdt(0,2,0)
  Bayer_to_Vid : Subsystem
  Buff_5x5 : Subsystem
  Calc_Kern : Subsystem
      settings: AttributesFormatString=|
      | ----------
      | op:1
      | ip:1
      | dp:on
  DlyMatch : Delay  DelayLength=2*C+2
  DlyMatch1 : Delay  DelayLength=2*C+2
  DlyMatch2 : Delay  DelayLength=2*C+2
  Get_Bayer : hdlsllib/HDL Operations/Bit Slice  lidx=7  ridx=0
      settings: SourceProductName=HDL Coder  SourceProductBaseCode=HD
  RGB_to_Vid : Subsystem
  Select_Pixel : Subsystem
      settings: AttributesFormatString=|
      | ----------
      | fh:on
  StateTracking : Subsystem
  Switch : Switch  Criteria=u2 ~= 0
      settings: AttributesFormatString=|
      | ----------
      | op:1
      | ip:1
  get_sof : Subsystem
      settings: AttributesFormatString=|
      | ----------
      | ip:1
  Video_o : Outport
  wires:
  Bayer_Phase/1 -> StateTracking/2(Bayer_Phase)
  Video_i/1 -> get_sof/1(Video_i)
  Buff_5x5/1(Dly_5x5) -> Calc_Kern/1(Dly_5x5)
  get_sof/2(Video_o) -> Get_Bayer/1
  get_sof/3(Rst) -> DlyMatch1/1
  DlyMatch1/1 -> StateTracking/1(Rst)
  DlyMatch/1 -> Bayer_to_Vid/2(Bayer), Select_Pixel/1(I)  "I_dly"
  Calc_Kern/1(Ir1b2) -> Select_Pixel/2(Ir1b2)
  Calc_Kern/2(Ir2b1) -> Select_Pixel/3(Ir2b1)
  Calc_Kern/3(Irb) -> Select_Pixel/4(Irb)
  Calc_Kern/4(Ig) -> Select_Pixel/5(Ig)
  StateTracking/1(state) -> Select_Pixel/6(State)
  Select_Pixel/1(R) -> RGB_to_Vid/2(R)
  Select_Pixel/2(G) -> RGB_to_Vid/3(G)
  Select_Pixel/3(B) -> RGB_to_Vid/4(B)
  Get_Bayer/1 -> DlyMatch/1, Buff_5x5/1(Pixel)
  get_sof/1(SoF) -> DlyMatch2/1
  DlyMatch2/1 -> Bayer_to_Vid/1(SoF), RGB_to_Vid/1(SoF)
  Switch/1 -> Video_o/1
  CFA_En/1 -> Switch/2
  RGB_to_Vid/1(Video_o) -> Switch/1
  Bayer_to_Vid/1(Video_o) -> Switch/3

== system ZynqBallTrackerFPGA/fpga_dut/GammaCorrection/Gama CorrectionCore ==
  R_i : Inport
  G_i : Inport  Port=2
  B_i : Inport  Port=3
  P : Inport  Port=4
  GammaApprox : Subsystem
      settings: AttributesFormatString=|
      | ----------
      | op:1
      | ip:1
      | dp:on
  RGBtoYcbCr : Subsystem
      settings: AttributesFormatString=|
      | ----------
      | op:1
      | ip:1
      | dp:on
  YCbCrtoRGB : Subsystem
      settings: AttributesFormatString=|
      | ----------
      | op:1
      | ip:1
      | dp:on
  R_o : Outport
  G_o : Outport  Port=2
  B_o : Outport  Port=3
  wires:
  RGBtoYcbCr/1(Y) -> GammaApprox/1(Y_i)
  GammaApprox/1(Y_o) -> YCbCrtoRGB/1(Y)
  P/1 -> GammaApprox/2(P)
  RGBtoYcbCr/3(Cr) -> YCbCrtoRGB/3(Cr)
  YCbCrtoRGB/2(G) -> G_o/1
  YCbCrtoRGB/3(B) -> B_o/1
  RGBtoYcbCr/2(Cb) -> YCbCrtoRGB/2(Cb)
  YCbCrtoRGB/1(R) -> R_o/1
  R_i/1 -> RGBtoYcbCr/1(R)
  B_i/1 -> RGBtoYcbCr/3(B)
  G_i/1 -> RGBtoYcbCr/2(G)

== system ZynqBallTrackerFPGA/fpga_dut/GammaCorrection/RGB_to_Vid ==
  SoF : Inport
  R : Inport  Port=2
  G : Inport  Port=3
  B : Inport  Port=4
  Bit Concat{,1..3} (4 alike) : hdlsllib/HDL Operations/Bit Concat  numInputs=2
      settings: SourceProductName=HDL Coder  SourceProductBaseCode=HD
  Constant : Constant  Value=0  OutDataTypeStr=fixdt(0,7,0)  SampleTime=-1
  Video_o : Outport
  wires:
  Bit Concat1/1 -> Bit Concat3/2
  SoF/1 -> Bit Concat/1
  R/1 -> Bit Concat1/1
  B/1 -> Bit Concat2/2
  G/1 -> Bit Concat2/1
  Bit Concat2/1 -> Bit Concat1/2
  Bit Concat/1 -> Video_o/1
  Constant/1 -> Bit Concat3/1
  Bit Concat3/1 -> Bit Concat/2

== system ZynqBallTrackerFPGA/fpga_dut/GammaCorrection/Vid_to_RGB ==
  Video_i : Inport
  Blue : hdlsllib/HDL Operations/Bit Slice  lidx=7  ridx=0
      settings: SourceProductName=HDL Coder  SourceProductBaseCode=HD
  Green : hdlsllib/HDL Operations/Bit Slice  lidx=15  ridx=8
      settings: SourceProductName=HDL Coder  SourceProductBaseCode=HD
  Red : hdlsllib/HDL Operations/Bit Slice  lidx=23  ridx=16
      settings: SourceProductName=HDL Coder  SourceProductBaseCode=HD
  SoF : hdlsllib/HDL Operations/Bit Slice  lidx=31  ridx=31
      settings: SourceProductName=HDL Coder  SourceProductBaseCode=HD
  SoF_o : Outport
  R_o : Outport  Port=2
  G_o : Outport  Port=3
  B_o : Outport  Port=4
  wires:
  Blue/1 -> B_o/1  "B"
  Video_i/1 -> SoF/1, Red/1, Green/1, Blue/1
  Red/1 -> R_o/1  "R"
  Green/1 -> G_o/1  "G"
  SoF/1 -> SoF_o/1

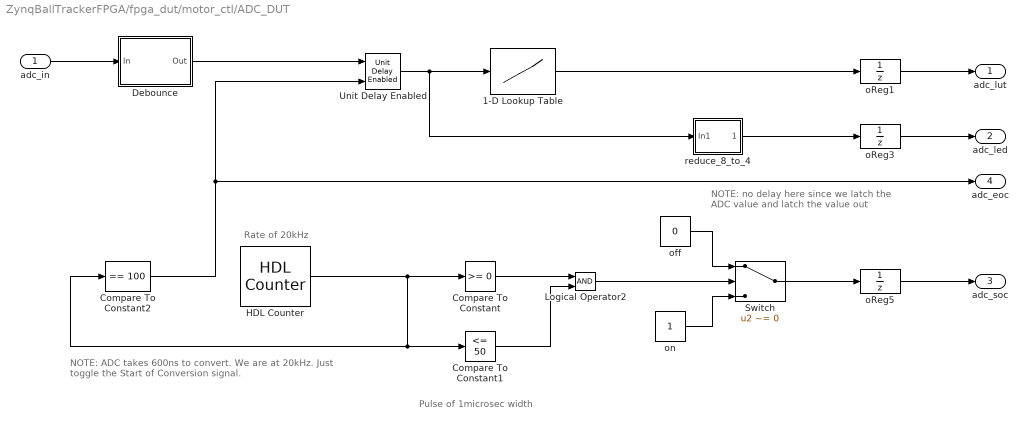
== system ZynqBallTrackerFPGA/fpga_dut/motor_ctl/ADC_DUT ==
  note: NOTE: no delay here since we latch the
      | ADC value and latch the value out
  note: Rate of 20kHz
  note: Pulse of 1microsec width
  note: NOTE: ADC takes 600ns to convert.  We are at 20kHz.
      | Just toggle the Start of Conversion signal.
  adc_in : Inport  OutDataTypeStr=uint8
  1-D Lookup Table : Lookup_n-D  NumberOfTableDimensions=1  BreakpointsForDimension1=[0:1:255]  IndexSearchMethod=Evenly spaced points  Table=[254:-2:-256]  TableDataTypeStr=Inherit: Inherit from 'Table data'  InterpMethod=Flat  DiagnosticForOutOfRangeInput=Error  OutDataTypeStr=fixdt(1,9,0)  RndMeth=Simplest  InputSameDT=on
  Compare To Constant : simulink/Logic and Bit Operations/Compare To Constant  relop=>=  const=0  OutDataTypeStr=boolean
  Compare To Constant1 : simulink/Logic and Bit Operations/Compare To Constant  relop=<=  const=50  OutDataTypeStr=boolean
  Compare To Constant2 : simulink/Logic and Bit Operations/Compare To Constant  relop===  const=100  OutDataTypeStr=boolean
  Debounce : Subsystem  TreatAsAtomicUnit=on  mask(Debounce){debounce_count=20}
      mask prompts: debounce_count "Debounce count"
      mask help: Number of consecutive samples before changing states.
  HDL Counter : hdlsllib/HDL Operations/HDL Counter  CountType=Count limited  CountInit=0  CountStep=1  CountMax=2500  CountFromType=Initial value  CountFrom=0  CountResetPort=off  CountLoadPort=off  CountEnbPort=off  CountDirPort=off  CountDataType=Unsigned  CountWordLen=12  CountFracLen=0  CountSampTime=-1
      settings: SourceProductName=HDL Coder  SourceProductBaseCode=HD
  Logical Operator2 : Logic  IconShape=distinctive  AllPortsSameDT=off  OutDataTypeStr=boolean
  Switch : Switch  Criteria=u2 ~= 0
  Unit Delay Enabled : simulink_need_slupdate/Unit Delay Enabled  vinit=5  tsamp=-1
      settings: SourceProductName=Simulink  SourceProductBaseCode=SL
  oReg1 : UnitDelay  SampleTime=-1
  oReg3 : UnitDelay  SampleTime=-1
  oReg5 : UnitDelay  SampleTime=-1
  off : Constant  Value=0  OutDataTypeStr=boolean  SampleTime=-1
  on : Constant  OutDataTypeStr=boolean  SampleTime=-1
  reduce_8_to_4 : Subsystem
  adc_lut : Outport
  adc_led : Outport  Port=2
  adc_soc : Outport  Port=3
  adc_eoc : Outport  Port=4
  wires:
  adc_in/1 -> Debounce/1(In)
  HDL Counter/1 -> Compare To Constant2/1, Compare To Constant1/1, Compare To Constant/1
  oReg1/1 -> adc_lut/1
  Compare To Constant/1 -> Logical Operator2/1
  oReg5/1 -> adc_soc/1
  Debounce/1(Out) -> Unit Delay Enabled/1
  Logical Operator2/1 -> Switch/2
  Compare To Constant1/1 -> Logical Operator2/2
  Unit Delay Enabled/1 -> reduce_8_to_4/1(In1), 1-D Lookup Table/1
  1-D Lookup Table/1 -> oReg1/1
  oReg3/1 -> adc_led/1
  off/1 -> Switch/1
  on/1 -> Switch/3
  Switch/1 -> oReg5/1
  Compare To Constant2/1 -> adc_eoc/1, Unit Delay Enabled/2
  reduce_8_to_4/1(Out1) -> oReg3/1

== system ZynqBallTrackerFPGA/fpga_dut/motor_ctl/PID_Controller ==
  des_pos : Inport  Interpolate=off
  act_pos : Inport  Port=2  Interpolate=off
  Kp : Inport  Port=3
  Ki : Inport  Port=4
  Kd : Inport  Port=5
  Abs : Abs
  Add : Sum  Inputs=+-
  Compare To Zero : simulink/Logic and Bit Operations/Compare To Zero  relop=>  OutDataTypeStr=boolean
  Data Type Conversion : DataTypeConversion  OutDataTypeStr=fixdt(0,9,0)
  PID_Controller_Programmable : Subsystem
  Sign : Signum
  controlsignal : Outport  InitialOutput=0
  polarity : Outport  Port=2  InitialOutput=0
  wires:
  Abs/1 -> Data Type Conversion/1  "ABS ERROR"
  Sign/1 -> Compare To Zero/1
  Compare To Zero/1 -> polarity/1  "SIGN"
  des_pos/1 -> Add/1  "DES_POS"
  act_pos/1 -> Add/2  "CURRENT_POS"
  PID_Controller_Programmable/1(controlsignal) -> Sign/1, Abs/1
  Ki/1 -> PID_Controller_Programmable/3(IGain)
  Kp/1 -> PID_Controller_Programmable/2(PGain)
  Kd/1 -> PID_Controller_Programmable/4(DGain)
  Data Type Conversion/1 -> controlsignal/1
  Add/1 -> PID_Controller_Programmable/1(error_delta)  "ERROR"

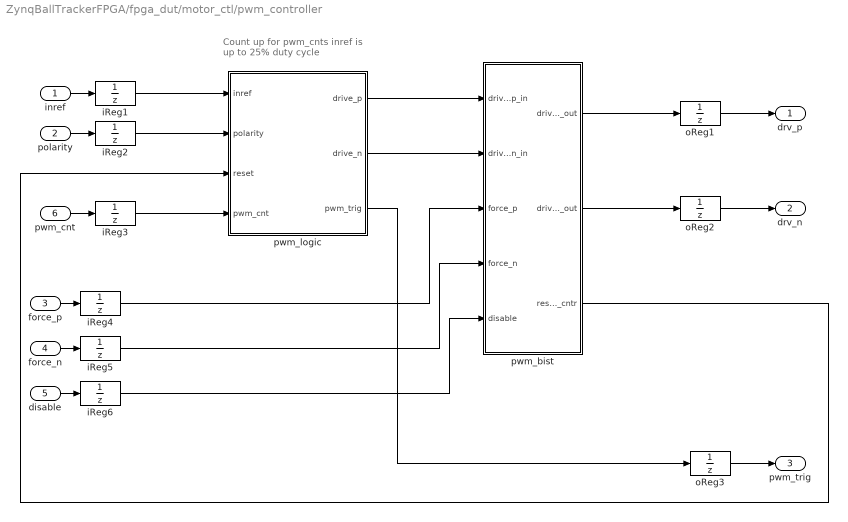
== system ZynqBallTrackerFPGA/fpga_dut/motor_ctl/pwm_controller ==
  note: Count up for pwm_cnts
      | inref is up to 25% duty cycle
  inref : Inport
  polarity : Inport  Port=2
  force_p : Inport  Port=3
  force_n : Inport  Port=4
  disable : Inport  Port=5
  pwm_cnt : Inport  Port=6
  iReg{1..6} (6 alike) : UnitDelay  SampleTime=-1
  oReg1 : UnitDelay  SampleTime=-1
  oReg2 : UnitDelay  SampleTime=-1
  oReg3 : UnitDelay  SampleTime=-1
  pwm_bist : Subsystem
  pwm_logic : Subsystem
  drv_p : Outport
  drv_n : Outport  Port=2
  pwm_trig : Outport  Port=3
  wires:
  iReg6/1 -> pwm_bist/5(disable)
  disable/1 -> iReg6/1
  oReg3/1 -> pwm_trig/1
  oReg2/1 -> drv_n/1
  oReg1/1 -> drv_p/1
  iReg5/1 -> pwm_bist/4(force_n)
  iReg4/1 -> pwm_bist/3(force_p)
  iReg2/1 -> pwm_logic/2(polarity)
  iReg1/1 -> pwm_logic/1(inref)
  pwm_bist/3(reset_cntr) -> pwm_logic/3(reset)
  pwm_logic/3(pwm_trig) -> oReg3/1
  force_n/1 -> iReg5/1
  force_p/1 -> iReg4/1
  pwm_logic/2(drive_n) -> pwm_bist/2(drive_n_in)
  pwm_logic/1(drive_p) -> pwm_bist/1(drive_p_in)
  polarity/1 -> iReg2/1
  pwm_bist/2(drive_n_out) -> oReg2/1
  inref/1 -> iReg1/1
  pwm_bist/1(drive_p_out) -> oReg1/1
  pwm_cnt/1 -> iReg3/1
  iReg3/1 -> pwm_logic/4(pwm_cnt)

== system ZynqBallTrackerFPGA/fpga_dut/BallTracker/FindCentroid/ROI ==
  BW_i : Inport
  x : Inport  Port=2
  y : Inport  Port=3
  xtarg : Inport  Port=4
  xthresh : Inport  Port=5
  ytarg : Inport  Port=6
  ythresh : Inport  Port=7
  Logical Operator : Logic  IconShape=distinctive  AllPortsSameDT=off  OutDataTypeStr=boolean
  Logical Operator1 : Logic  IconShape=distinctive  AllPortsSameDT=off  OutDataTypeStr=boolean
      settings: AttributesFormatString=|
      | ----------
      | op:1
      | ip:1
  abserr : Abs
  abserr1 : Abs
  err : Sum  Inputs=+-
      settings: AttributesFormatString=|
      | ----------
      | op:1
      | ip:1
  err1 : Sum  Inputs=+-
      settings: AttributesFormatString=|
      | ----------
      | op:1
      | ip:1
  lt : RelationalOperator  Operator=<  OutDataTypeStr=boolean  RndMeth=Nearest
      settings: AttributesFormatString=|
      | ----------
      | op:1
      | ip:1
  lt1 : RelationalOperator  Operator=<  OutDataTypeStr=boolean  RndMeth=Nearest
      settings: AttributesFormatString=|
      | ----------
      | op:1
      | ip:1
  BW_o : Outport
  wires:
  xtarg/1 -> err/2
  err/1 -> abserr/1  "Xerr"
  abserr/1 -> lt/1  "aXerr"
  xthresh/1 -> lt/2
  lt/1 -> Logical Operator/1  "Xok"
  x/1 -> err/1
  ytarg/1 -> err1/2
  err1/1 -> abserr1/1  "Yerr"
  abserr1/1 -> lt1/1  "aYerr"
  ythresh/1 -> lt1/2
  lt1/1 -> Logical Operator/2  "Yok"
  y/1 -> err1/1
  Logical Operator/1 -> Logical Operator1/2
  BW_i/1 -> Logical Operator1/1
  Logical Operator1/1 -> BW_o/1

== system ZynqBallTrackerFPGA/fpga_dut/BallTracker/FindCentroid/TimingSubsystem ==
  Rst : Inport
  Compare To Constant : simulink/Logic and Bit Operations/Compare To Constant  relop===  const=R-1  OutDataTypeStr=boolean
  Compare To Constant1 : simulink/Logic and Bit Operations/Compare To Constant  relop===  const=C-1  OutDataTypeStr=boolean
  Logical Operator : Logic  IconShape=distinctive  AllPortsSameDT=off  OutDataTypeStr=boolean
  Pix_Pos : Subsystem
  en : Constant  Value=true  SampleTime=-1
  Y : Outport
  X : Outport  Port=2
  LastPix : Outport  Port=3
  wires:
  Pix_Pos/1(Column) -> Compare To Constant1/1, X/1
  Pix_Pos/2(Row) -> Compare To Constant/1, Y/1
  Rst/1 -> Pix_Pos/2(Rst)
  en/1 -> Pix_Pos/1(Vld)
  Compare To Constant1/1 -> Logical Operator/1
  Compare To Constant/1 -> Logical Operator/2
  Logical Operator/1 -> LastPix/1

== system ZynqBallTrackerFPGA/fpga_dut/BallTracker/FindCentroid/accum_to_pos ==
  y_accum : Inport
  x_accum : Inport  Port=2
  npoints : Inport  Port=3
  Data Type Conversion : DataTypeConversion  OutDataTypeStr=uint32  SaturateOnIntegerOverflow=on  RndMeth=Zero
      settings: AttributesFormatString=|
      | ----------
      | op:1
      | ip:1
  Data Type Conversion1 : DataTypeConversion  OutDataTypeStr=uint32  SaturateOnIntegerOverflow=on  RndMeth=Zero
      settings: AttributesFormatString=|
      | ----------
      | op:1
      | ip:1
  recip : Product  Inputs=/  OutDataTypeStr=fixdt(0,22,22)  SaturateOnIntegerOverflow=on  RndMeth=Zero
      settings: AttributesFormatString=|
      | ----------
      | op:2
      | ip:2
  x_pos : Product
      settings: AttributesFormatString=|
      | ----------
      | op:3
      | ip:2
  y_pos : Product
      settings: AttributesFormatString=|
      | ----------
      | op:3
      | ip:2
  y_o : Outport
  x_o : Outport  Port=2
  wires:
  x_pos/1 -> Data Type Conversion1/1
  Data Type Conversion/1 -> y_o/1
  y_pos/1 -> Data Type Conversion/1
  Data Type Conversion1/1 -> x_o/1
  npoints/1 -> recip/1
  recip/1 -> y_pos/2, x_pos/2
  x_accum/1 -> x_pos/1
  y_accum/1 -> y_pos/1

== system ZynqBallTrackerFPGA/fpga_dut/BallTracker/FindCentroid/npts_accum ==
  Inc : Inport
  Rst : Inport  Port=2
  En : Inport  Port=3
  Add : Sum  OutDataTypeStr=fixdt(0,ceil(log2(MaxVal)),0)  RndMeth=Zero  SaturateOnIntegerOverflow=on
  Logical Operator : Logic  Operator=OR  IconShape=distinctive  AllPortsSameDT=off  OutDataTypeStr=boolean
  Switch : Switch  Criteria=u2 ~= 0
  Unit Delay Enabled : simulink_need_slupdate/Unit Delay Enabled  vinit=fi(0,0,32,0)  tsamp=-1
      settings: SourceProductName=Simulink  SourceProductBaseCode=SL
  zero : Constant  Value=0  OutDataTypeStr=Inherit: Inherit via back propagation  SampleTime=-1
  Cnt : Outport
  wires:
  En/1 -> Logical Operator/2
  Rst/1 -> Logical Operator/1, Switch/2
  zero/1 -> Switch/1
  Add/1 -> Switch/3
  Logical Operator/1 -> Unit Delay Enabled/2
  Switch/1 -> Unit Delay Enabled/1
  Inc/1 -> Add/2  "xinc"
  Unit Delay Enabled/1 -> Add/1, Cnt/1

== system ZynqBallTrackerFPGA/fpga_dut/BallTracker/FindCentroid/x_accum ==
  Inc : Inport
  Rst : Inport  Port=2
  En : Inport  Port=3
  Add : Sum  OutDataTypeStr=fixdt(0,ceil(log2(MaxVal)),0)  RndMeth=Zero  SaturateOnIntegerOverflow=on
  Logical Operator : Logic  Operator=OR  IconShape=distinctive  AllPortsSameDT=off  OutDataTypeStr=boolean
  Switch : Switch  Criteria=u2 ~= 0
  Unit Delay Enabled : simulink_need_slupdate/Unit Delay Enabled  vinit=fi(0,0,32,0)  tsamp=-1
      settings: SourceProductName=Simulink  SourceProductBaseCode=SL
  zero : Constant  Value=0  OutDataTypeStr=Inherit: Inherit via back propagation  SampleTime=-1
  Cnt : Outport
  wires:
  Unit Delay Enabled/1 -> Cnt/1, Add/1
  Inc/1 -> Add/2  "xinc"
  Switch/1 -> Unit Delay Enabled/1
  Logical Operator/1 -> Unit Delay Enabled/2
  Add/1 -> Switch/3
  zero/1 -> Switch/1
  Rst/1 -> Switch/2, Logical Operator/1
  En/1 -> Logical Operator/2
